simulink model "threeDiskOscillatorRig_v3_1"  (R2024b)
settings: Solver=VariableStepAuto  StartTime=0.0  StopTime=simTime  RelTol=1e-3
values from neighbouring files (symbols this model uses):
  h = double(vpasolve(eq_1,gg))    [threeDiskOscillator.m]
  mu_0 = 0    [threeDiskOscillator.m]
  r2 = testout.r1.signals.values(:,2)    [threeDiskOscillator.m]
  T_s = 4e-3    (= 0.004)    [threeDiskOscillator.m]
undefined symbols (not defined in the file or in its folder): M_window, var
settings Model: Creator=nicol  LastModifiedBy=nicol

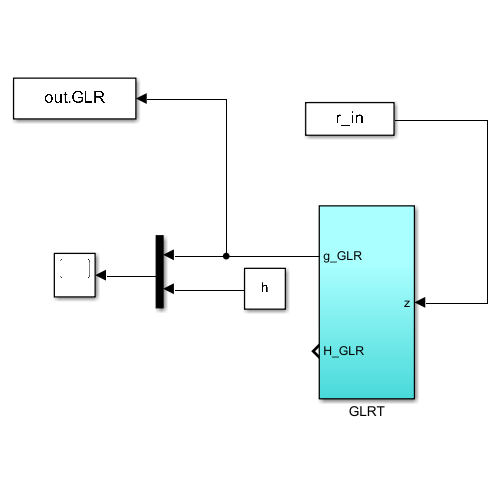
[thumbnail: Simulink's stored preview of the top-level diagram]
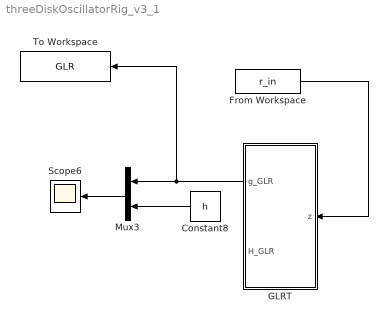
== system threeDiskOscillatorRig_v3_1 ==
  Constant8 : Constant  Value=h
  From Workspace : FromWorkspace  VariableName=r_in
  GLRT : Subsystem
  Mux3 : Mux  Inputs=2
  Scope6 : Scope
  To Workspace : ToWorkspace  VariableName=GLR  SaveFormat=Timeseries  SampleTime=T_s
  wires:
  GLRT/1(g_GLR) -> To Workspace/1, Mux3/1
  Constant8/1 -> Mux3/2
  Mux3/1 -> Scope6/1
  From Workspace/1 -> GLRT/1(z)

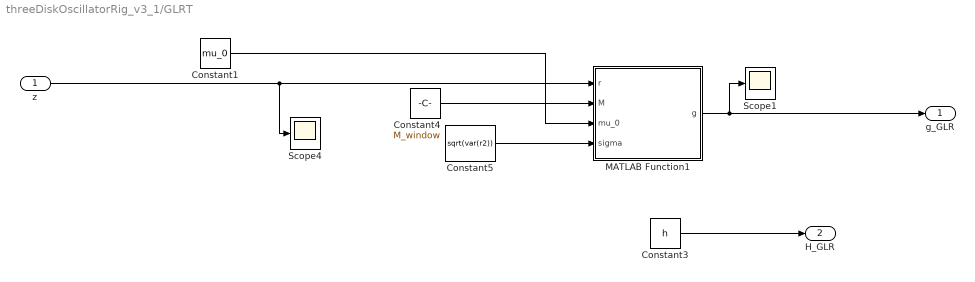
== system threeDiskOscillatorRig_v3_1/GLRT ==
  z : Inport
  Constant1 : Constant  Value=mu_0
  Constant3 : Constant  Value=h
  Constant4 : Constant  Value=M_window
  Constant5 : Constant  Value=sqrt(var(r2))
  MATLAB Function1 : MATLAB Function  TreatAsAtomicUnit=on
  Scope1 : Scope
  Scope4 : Scope
  g_GLR : Outport  VectorParamsAs1DForOutWhenUnconnected=off
  H_GLR : Outport  Port=2  VectorParamsAs1DForOutWhenUnconnected=off
  wires:
  Constant5/1 -> MATLAB Function1/4(sigma)
  Constant1/1 -> MATLAB Function1/3(mu_0)
  Constant4/1 -> MATLAB Function1/2(M)
  MATLAB Function1/1(g) -> g_GLR/1, Scope1/1
  z/1 -> Scope4/1, MATLAB Function1/1(r)
  Constant3/1 -> H_GLR/1

== matlab function threeDiskOscillatorRig_v3_1/GLRT/MATLAB Function1 ==
  settings: updateMethod=DISCRETE
  data: r input; M input; mu_0 input; sigma input; g output
function g  = GLR(r,M,mu_0,sigma)
%GLR 
%M =initial guess of window size
%mu_0 = mean value when no fault occured 
%sigma = standard deviation of residual

  persistent buffer mu_1 idx
  g = 0;
 
 %initialization at start
 if (isempty(buffer))
    buffer = zeros(1, M);
    %g = 0;      
    mu_1 = 0;   
    idx = 0;    
 end

%right shift buffer which keeps the lates M samples: 
buffer = [r, buffer(1:end-1)];   
if length(buffer) > M
    buffer = buffer(1:M);
end

% Compute GLR When M samples are stores in the buffer
if (length(buffer) == M)
    S = zeros(M, 1);  % Define the log-likelihood ratio
    z = buffer;       % extract the residual samples inside the window 
    for j = 1:M       % Iterate for all the time instants of the window
        sum_sq = 0;
        for i = j:M
            sum_sq = sum_sq + (z(i) - mu_0);
        end
        S(j) = sum_sq^2 / ((M - j + 1) * 2 * sigma^2);
    end
    
    % Find maximum GLR statistic and corresponding index
    [g, idx] = max(S); 
    mu_1= sum(buffer(idx:end)) / (M - idx + 1);
else 
    j=0
    z=buffer;
    sum_sq=0;
    S = zeros(M, 1); 

end

end
